simulink model "watertankscheduling"  (R2021a)
settings: Solver=VariableStepAuto  StartTime=0.0  StopTime=T_max  RelTol=1e-3
undefined symbols (not defined in the file or in its folder): A_tank, h0, H_max
libraries: rllib x1
settings Model: Creator=The MathWorks, Inc.  LastModifiedBy=prash
settings SolverCC: AlgebraicLoopSolver=TrustRegion
settings DebuggingCC: SFMachineParentedDataDiag=warning

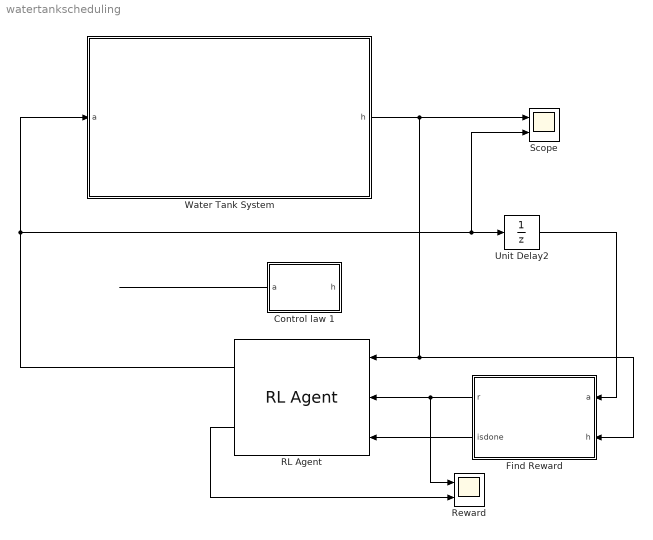
== system watertankscheduling ==
  Control law 1 : MATLAB Function  TreatAsAtomicUnit=on  SystemSampleTime=.1
  Find Reward : MATLAB Function  TreatAsAtomicUnit=on
  RL Agent : rllib/RL Agent  Agent=agent  ExternalActionAsInput=off  ProvideCumRwd=on  TreatAsDirectFeedthrough=on
  Reward : Scope  NumInputPorts=2
  Scope : Scope  NumInputPorts=2
  Unit Delay2 : UnitDelay  SampleTime=-1  HasFrameUpgradeWarning=on
  Water Tank System : Subsystem
      mask Display: image('$imagefile'); % Use "Edit Image" on toolstrip to change.
  wires:
  Control law 1/1(a) -> ?
  Find Reward/2(isdone) -> RL Agent/3
  Unit Delay2/1 -> Find Reward/1(a)
  Find Reward/1(r) -> RL Agent/2, Reward/1
  RL Agent/2 -> Reward/2
  RL Agent/1 -> Water Tank System/1(a), Scope/2, Unit Delay2/1
  Water Tank System/1(h) -> Scope/1, Find Reward/2(h), RL Agent/1

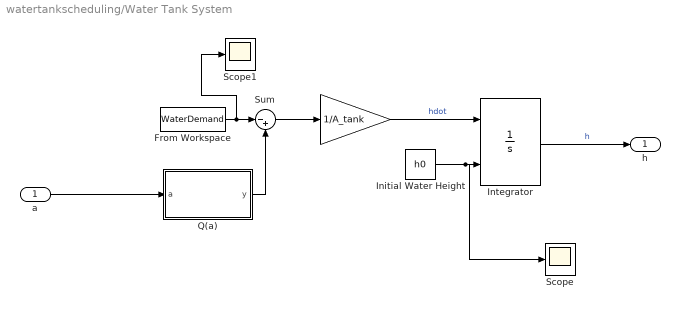
== system watertankscheduling/Water Tank System ==
  a : Inport
  " " : Gain  Gain=1/A_tank
  From Workspace : FromWorkspace  VariableName=WaterDemand  SampleTime=.1
  Initial Water Height : Constant  Value=h0
  Integrator : Integrator  InitialConditionSource=external  LimitOutput=on  UpperSaturationLimit=H_max  LowerSaturationLimit=0
  Q(a) : MATLAB Function  TreatAsAtomicUnit=on
  Scope : Scope
  Scope1 : Scope
  Sum : Sum  Inputs=|-+
  h : Outport
  wires:
  From Workspace/1 -> Scope1/1, Sum/1
  " "/1 -> Integrator/1  "hdot"
  a/1 -> Q(a)/1(a)
  Integrator/1 -> h/1  "h"
  Sum/1 -> " "/1
  Q(a)/1(y) -> Sum/2
  Initial Water Height/1 -> Scope/1, Integrator/2

== matlab function watertankscheduling/Control law 1 ==
  data: h input; a output
function a = fcn(h)

break1 = 4.5;
break2 =3.5;

a = 0;
if h<6.8 && h>=break1
    a = 1;
elseif h<break1 && h>=break2
    a = 2;
elseif h<break2
    a = 3;
end

== matlab function watertankscheduling/Water Tank System/Q(a) ==
  data: a input; y output
function y = fcn(a)
% y: flow rate m^3/hr
% a: number of active pumps
switch int8(a)
    case 0
        y = 0;
    case 1
        y = 164;
    case 2
        y = 279;
    case 3
        y = 344;
    otherwise
        error('Invalid input')
end

== matlab function watertankscheduling/Find Reward ==
  data: a input; h input; r output; isdone output
function [r,isdone] = fcn(a,h)
H_max = 7;
NormalizeTerm = 13.0; %3.5
isdone = false;
if h>=(H_max-0.1)
    r = -a - 10;
elseif h>0.1  &&  h<(H_max-0.1)
    r = -a;
else
    r = -a - 10;
end

r = r/NormalizeTerm;    
% H_max = 7;
% NormalizeTerm = 5.0; %3.5
% isdone = false;
% if h>=(H_max-.1)
%     r = -a - 1;
% elseif h>0.1
%     r = -a;
% else
%     r = -a - 2;
% end
% 
% r = r/NormalizeTerm;
